simulink model "VIPStateCtrl"  (R2018b)
settings: Solver=FixedStepDiscrete  StartTime=0.0  StopTime=10.0  FixedStep=0.01  RelTol=1e-3
settings Model: Creator=sn2xws  LastModifiedBy=sn2xws
settings DataIOCC: SaveFormat=StructureWithTime
settings OptimizationCC: DefaultParameterBehavior=Inlined  EnhancedBackFolding=on  PassReuseOutputArgsAs=Individual arguments  ZeroExternalMemoryAtStartup=off  ZeroInternalMemoryAtStartup=off  OptimizeBlockOrder=speed  DifferentSizesBufferReuse=on  OptimizationCustomize=off
settings DebuggingCC: ParameterTunabilityLossMsg=error
settings ModelReferenceCC: ModelReferenceNumInstancesAllowed=Single
settings SFSimCC: MATLABDynamicMemAlloc=off
settings RTWCC: SystemTargetFile=autosar.tlc  GenCodeOnly=on  TemplateMakefile=ert_default_tmf  Description=AUTOSAR  GenerateReport=on  IncludeHyperlinkInReport=on  LaunchReport=on  GenerateTraceInfo=on  GenerateTraceReport=on  GenerateTraceReportSl=on  GenerateTraceReportSf=on  GenerateTraceReportEml=on
settings CodeAppCC: ForceParamTrailComments=on  IgnoreCustomStorageClasses=off  OperatorAnnotations=on  SimulinkDataObjDesc=on  SFDataObjDesc=on  InsertBlockDesc=on
settings STFCustomTargetCC: TargetLangStandard=C99 (ISO)  MultiwordLength=256  ParMdlRefBuildCompliant=on  CompOptLevelCompliant=on  IncludeMdlTerminateFcn=off  CombineOutputUpdateFcns=on  SuppressErrorStatus=on  ERTCustomFileBanners=on  SupportNonFinite=off  SupportComplex=off  SupportContinuousTime=off  SupportNonInlinedSFcns=off  RemoveResetFunc=on  MATLABClassNameForMDSCustomization=Simulink.SoftwareTarget.ERTCustomization  AutosarCompliant=on  UseToolchainInfoCompliant=on  LookupTableObjectStructAxisOrder=2,1,3,4,...  LUTObjectStructOrderEvenSpacing=Size,Table,Breakpoints  SystemTargetFile=autosar.tlc
settings ERTTargetCC: TargetLangStandard=C99 (ISO)  ConcurrentExecutionCompliant=off  IncludeMdlTerminateFcn=off  SuppressErrorStatus=on  SupportNonFinite=off  SupportComplex=off  ModelStepFunctionPrototypeControlCompliant=off  CPPClassGenCompliant=off  AutosarCompliant=on  LookupTableObjectStructAxisOrder=2,1,3,4,...  LUTObjectStructOrderEvenSpacing=Size,Table,Breakpoints  InlinedParameterPlacement=NonHierarchical  ERTCustomFileTemplate=example_file_process.tlc

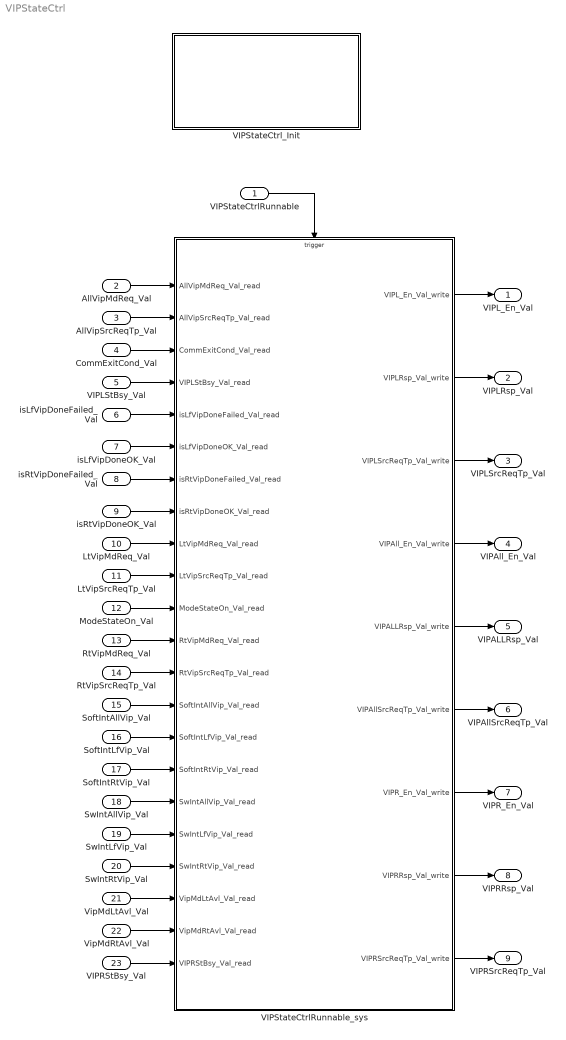
== system VIPStateCtrl ==
  VIPStateCtrlRunnable : Inport  SampleTime=0.01  OutputFunctionCall=on
  AllVipMdReq_Val : Inport  Port=2  OutDataTypeStr=boolean  PortDimensions=1
  AllVipSrcReqTp_Val : Inport  Port=3  OutDataTypeStr=Enum: SrcReqTp1  PortDimensions=1
  CommExitCond_Val : Inport  Port=4  OutDataTypeStr=boolean  PortDimensions=1
  VIPLStBsy_Val : Inport  Port=5  OutDataTypeStr=boolean  PortDimensions=1
  isLfVipDoneFailed_Val : Inport  Port=6  OutDataTypeStr=boolean  PortDimensions=1
  isLfVipDoneOK_Val : Inport  Port=7  OutDataTypeStr=boolean  PortDimensions=1
  isRtVipDoneFailed_Val : Inport  Port=8  OutDataTypeStr=boolean  PortDimensions=1
  isRtVipDoneOK_Val : Inport  Port=9  OutDataTypeStr=boolean  PortDimensions=1
  LtVipMdReq_Val : Inport  Port=10  OutDataTypeStr=boolean  PortDimensions=1
  LtVipSrcReqTp_Val : Inport  Port=11  OutDataTypeStr=Enum: SrcReqTp1  PortDimensions=1
  ModeStateOn_Val : Inport  Port=12  OutDataTypeStr=boolean  PortDimensions=1
  RtVipMdReq_Val : Inport  Port=13  OutDataTypeStr=boolean  PortDimensions=1
  RtVipSrcReqTp_Val : Inport  Port=14  OutDataTypeStr=Enum: SrcReqTp1  PortDimensions=1
  SoftIntAllVip_Val : Inport  Port=15  OutDataTypeStr=IntEnable  PortDimensions=1
  SoftIntLfVip_Val : Inport  Port=16  OutDataTypeStr=IntEnable  PortDimensions=1
  SoftIntRtVip_Val : Inport  Port=17  OutDataTypeStr=IntEnable  PortDimensions=1
  SwIntAllVip_Val : Inport  Port=18  OutDataTypeStr=IntEnable  PortDimensions=1
  SwIntLfVip_Val : Inport  Port=19  OutDataTypeStr=IntEnable  PortDimensions=1
  SwIntRtVip_Val : Inport  Port=20  OutDataTypeStr=IntEnable  PortDimensions=1
  VipMdLtAvl_Val : Inport  Port=21  OutDataTypeStr=boolean  PortDimensions=1
  VipMdRtAvl_Val : Inport  Port=22  OutDataTypeStr=boolean  PortDimensions=1
  VIPRStBsy_Val : Inport  Port=23  OutDataTypeStr=boolean  PortDimensions=1
  VIPStateCtrlRunnable_sys : Subsystem
  VIPStateCtrl_Init : Subsystem
  VIPL_En_Val : Outport  OutDataTypeStr=boolean  PortDimensions=1
  VIPLRsp_Val : Outport  Port=2  OutDataTypeStr=Enum: MdRspLocal1  PortDimensions=1
  VIPLSrcReqTp_Val : Outport  Port=3  OutDataTypeStr=Enum: SrcReqTp1  PortDimensions=1
  VIPAll_En_Val : Outport  Port=4  OutDataTypeStr=boolean  PortDimensions=1
  VIPALLRsp_Val : Outport  Port=5  OutDataTypeStr=Enum: MdRspLocal1  PortDimensions=1
  VIPAllSrcReqTp_Val : Outport  Port=6  OutDataTypeStr=Enum: SrcReqTp1  PortDimensions=1
  VIPR_En_Val : Outport  Port=7  OutDataTypeStr=boolean  PortDimensions=1
  VIPRRsp_Val : Outport  Port=8  OutDataTypeStr=Enum: MdRspLocal1  PortDimensions=1
  VIPRSrcReqTp_Val : Outport  Port=9  OutDataTypeStr=Enum: SrcReqTp1  PortDimensions=1
  wires:
  AllVipMdReq_Val/1 -> VIPStateCtrlRunnable_sys/1(AllVipMdReq_Val_read)
  AllVipSrcReqTp_Val/1 -> VIPStateCtrlRunnable_sys/2(AllVipSrcReqTp_Val_read)
  CommExitCond_Val/1 -> VIPStateCtrlRunnable_sys/3(CommExitCond_Val_read)
  VIPLStBsy_Val/1 -> VIPStateCtrlRunnable_sys/4(VIPLStBsy_Val_read)
  isLfVipDoneFailed_Val/1 -> VIPStateCtrlRunnable_sys/5(isLfVipDoneFailed_Val_read)
  isLfVipDoneOK_Val/1 -> VIPStateCtrlRunnable_sys/6(isLfVipDoneOK_Val_read)
  isRtVipDoneFailed_Val/1 -> VIPStateCtrlRunnable_sys/7(isRtVipDoneFailed_Val_read)
  isRtVipDoneOK_Val/1 -> VIPStateCtrlRunnable_sys/8(isRtVipDoneOK_Val_read)
  LtVipMdReq_Val/1 -> VIPStateCtrlRunnable_sys/9(LtVipMdReq_Val_read)
  LtVipSrcReqTp_Val/1 -> VIPStateCtrlRunnable_sys/10(LtVipSrcReqTp_Val_read)
  ModeStateOn_Val/1 -> VIPStateCtrlRunnable_sys/11(ModeStateOn_Val_read)
  RtVipMdReq_Val/1 -> VIPStateCtrlRunnable_sys/12(RtVipMdReq_Val_read)
  RtVipSrcReqTp_Val/1 -> VIPStateCtrlRunnable_sys/13(RtVipSrcReqTp_Val_read)
  SoftIntAllVip_Val/1 -> VIPStateCtrlRunnable_sys/14(SoftIntAllVip_Val_read)
  SoftIntLfVip_Val/1 -> VIPStateCtrlRunnable_sys/15(SoftIntLfVip_Val_read)
  SoftIntRtVip_Val/1 -> VIPStateCtrlRunnable_sys/16(SoftIntRtVip_Val_read)
  SwIntAllVip_Val/1 -> VIPStateCtrlRunnable_sys/17(SwIntAllVip_Val_read)
  SwIntLfVip_Val/1 -> VIPStateCtrlRunnable_sys/18(SwIntLfVip_Val_read)
  SwIntRtVip_Val/1 -> VIPStateCtrlRunnable_sys/19(SwIntRtVip_Val_read)
  VipMdLtAvl_Val/1 -> VIPStateCtrlRunnable_sys/20(VipMdLtAvl_Val_read)
  VipMdRtAvl_Val/1 -> VIPStateCtrlRunnable_sys/21(VipMdRtAvl_Val_read)
  VIPRStBsy_Val/1 -> VIPStateCtrlRunnable_sys/22(VIPRStBsy_Val_read)
  VIPStateCtrlRunnable_sys/1(VIPL_En_Val_write) -> VIPL_En_Val/1
  VIPStateCtrlRunnable_sys/2(VIPLRsp_Val_write) -> VIPLRsp_Val/1
  VIPStateCtrlRunnable_sys/3(VIPLSrcReqTp_Val_write) -> VIPLSrcReqTp_Val/1
  VIPStateCtrlRunnable_sys/4(VIPAll_En_Val_write) -> VIPAll_En_Val/1
  VIPStateCtrlRunnable_sys/5(VIPALLRsp_Val_write) -> VIPALLRsp_Val/1
  VIPStateCtrlRunnable_sys/6(VIPAllSrcReqTp_Val_write) -> VIPAllSrcReqTp_Val/1
  VIPStateCtrlRunnable_sys/7(VIPR_En_Val_write) -> VIPR_En_Val/1
  VIPStateCtrlRunnable_sys/8(VIPRRsp_Val_write) -> VIPRRsp_Val/1
  VIPStateCtrlRunnable_sys/9(VIPRSrcReqTp_Val_write) -> VIPRSrcReqTp_Val/1
  VIPStateCtrlRunnable/1 -> VIPStateCtrlRunnable_sys/Trigger

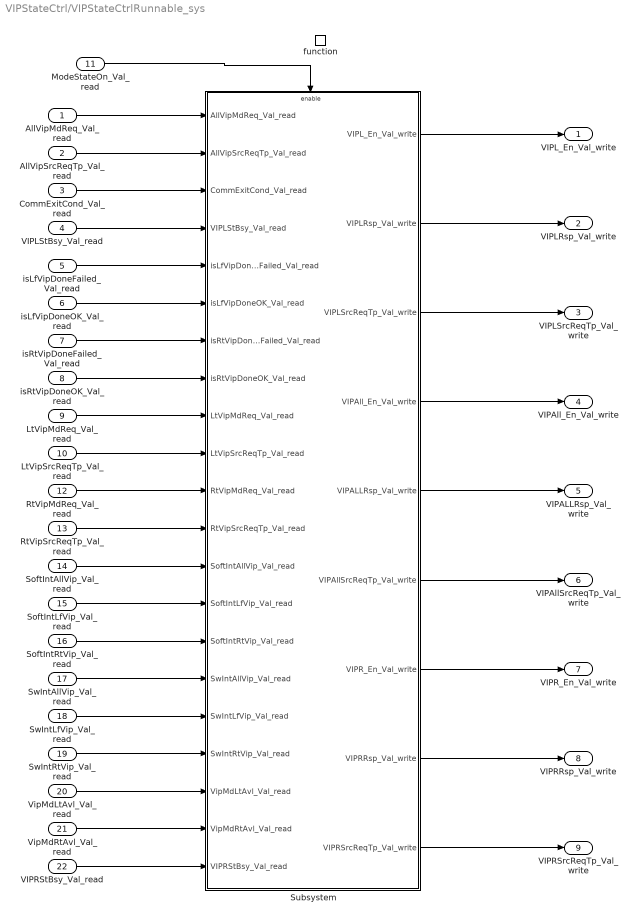
== system VIPStateCtrl/VIPStateCtrlRunnable_sys ==
  AllVipMdReq_Val_read : Inport
  AllVipSrcReqTp_Val_read : Inport  Port=2
  CommExitCond_Val_read : Inport  Port=3
  VIPLStBsy_Val_read : Inport  Port=4
  isLfVipDoneFailed_Val_read : Inport  Port=5
  isLfVipDoneOK_Val_read : Inport  Port=6
  isRtVipDoneFailed_Val_read : Inport  Port=7
  isRtVipDoneOK_Val_read : Inport  Port=8
  LtVipMdReq_Val_read : Inport  Port=9
  LtVipSrcReqTp_Val_read : Inport  Port=10
  ModeStateOn_Val_read : Inport  Port=11
  RtVipMdReq_Val_read : Inport  Port=12
  RtVipSrcReqTp_Val_read : Inport  Port=13
  SoftIntAllVip_Val_read : Inport  Port=14
  SoftIntLfVip_Val_read : Inport  Port=15
  SoftIntRtVip_Val_read : Inport  Port=16
  SwIntAllVip_Val_read : Inport  Port=17
  SwIntLfVip_Val_read : Inport  Port=18
  SwIntRtVip_Val_read : Inport  Port=19
  VipMdLtAvl_Val_read : Inport  Port=20
  VipMdRtAvl_Val_read : Inport  Port=21
  VIPRStBsy_Val_read : Inport  Port=22
  function : TriggerPort  TriggerType=function-call  VariantControl=(inherit)  SampleTimeType=periodic  SampleTime=-1
  Subsystem : Subsystem
  VIPL_En_Val_write : Outport
      settings: EnsureOutportIsVirtual=on
  VIPLRsp_Val_write : Outport  Port=2
      settings: EnsureOutportIsVirtual=on
  VIPLSrcReqTp_Val_write : Outport  Port=3
      settings: EnsureOutportIsVirtual=on
  VIPAll_En_Val_write : Outport  Port=4
      settings: EnsureOutportIsVirtual=on
  VIPALLRsp_Val_write : Outport  Port=5
      settings: EnsureOutportIsVirtual=on
  VIPAllSrcReqTp_Val_write : Outport  Port=6
      settings: EnsureOutportIsVirtual=on
  VIPR_En_Val_write : Outport  Port=7
      settings: EnsureOutportIsVirtual=on
  VIPRRsp_Val_write : Outport  Port=8
      settings: EnsureOutportIsVirtual=on
  VIPRSrcReqTp_Val_write : Outport  Port=9
      settings: EnsureOutportIsVirtual=on
  wires:
  ModeStateOn_Val_read/1 -> Subsystem/Enable
  AllVipMdReq_Val_read/1 -> Subsystem/1(AllVipMdReq_Val_read)
  AllVipSrcReqTp_Val_read/1 -> Subsystem/2(AllVipSrcReqTp_Val_read)
  CommExitCond_Val_read/1 -> Subsystem/3(CommExitCond_Val_read)
  VIPLStBsy_Val_read/1 -> Subsystem/4(VIPLStBsy_Val_read)
  isLfVipDoneFailed_Val_read/1 -> Subsystem/5(isLfVipDoneFailed_Val_read)
  isLfVipDoneOK_Val_read/1 -> Subsystem/6(isLfVipDoneOK_Val_read)
  isRtVipDoneFailed_Val_read/1 -> Subsystem/7(isRtVipDoneFailed_Val_read)
  isRtVipDoneOK_Val_read/1 -> Subsystem/8(isRtVipDoneOK_Val_read)
  LtVipMdReq_Val_read/1 -> Subsystem/9(LtVipMdReq_Val_read)
  LtVipSrcReqTp_Val_read/1 -> Subsystem/10(LtVipSrcReqTp_Val_read)
  RtVipMdReq_Val_read/1 -> Subsystem/11(RtVipMdReq_Val_read)
  RtVipSrcReqTp_Val_read/1 -> Subsystem/12(RtVipSrcReqTp_Val_read)
  SoftIntAllVip_Val_read/1 -> Subsystem/13(SoftIntAllVip_Val_read)
  SoftIntLfVip_Val_read/1 -> Subsystem/14(SoftIntLfVip_Val_read)
  SoftIntRtVip_Val_read/1 -> Subsystem/15(SoftIntRtVip_Val_read)
  SwIntAllVip_Val_read/1 -> Subsystem/16(SwIntAllVip_Val_read)
  SwIntLfVip_Val_read/1 -> Subsystem/17(SwIntLfVip_Val_read)
  SwIntRtVip_Val_read/1 -> Subsystem/18(SwIntRtVip_Val_read)
  VipMdLtAvl_Val_read/1 -> Subsystem/19(VipMdLtAvl_Val_read)
  VipMdRtAvl_Val_read/1 -> Subsystem/20(VipMdRtAvl_Val_read)
  VIPRStBsy_Val_read/1 -> Subsystem/21(VIPRStBsy_Val_read)
  Subsystem/1(VIPL_En_Val_write) -> VIPL_En_Val_write/1
  Subsystem/2(VIPLRsp_Val_write) -> VIPLRsp_Val_write/1
  Subsystem/3(VIPLSrcReqTp_Val_write) -> VIPLSrcReqTp_Val_write/1
  Subsystem/4(VIPAll_En_Val_write) -> VIPAll_En_Val_write/1
  Subsystem/5(VIPALLRsp_Val_write) -> VIPALLRsp_Val_write/1
  Subsystem/6(VIPAllSrcReqTp_Val_write) -> VIPAllSrcReqTp_Val_write/1
  Subsystem/7(VIPR_En_Val_write) -> VIPR_En_Val_write/1
  Subsystem/8(VIPRRsp_Val_write) -> VIPRRsp_Val_write/1
  Subsystem/9(VIPRSrcReqTp_Val_write) -> VIPRSrcReqTp_Val_write/1

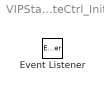
== system VIPStateCtrl/VIPStateCtrl_Init ==
  Event Listener : EventListener  EventName=reset

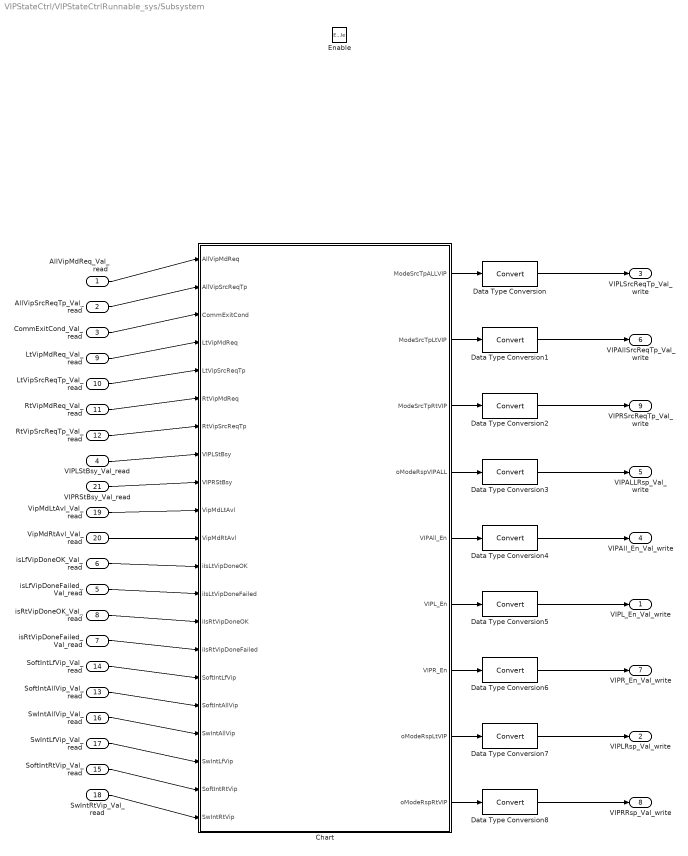
== system VIPStateCtrl/VIPStateCtrlRunnable_sys/Subsystem ==
  AllVipMdReq_Val_read : Inport
  AllVipSrcReqTp_Val_read : Inport  Port=2
  CommExitCond_Val_read : Inport  Port=3
  VIPLStBsy_Val_read : Inport  Port=4
  isLfVipDoneFailed_Val_read : Inport  Port=5
  isLfVipDoneOK_Val_read : Inport  Port=6
  isRtVipDoneFailed_Val_read : Inport  Port=7
  isRtVipDoneOK_Val_read : Inport  Port=8
  LtVipMdReq_Val_read : Inport  Port=9
  LtVipSrcReqTp_Val_read : Inport  Port=10
  RtVipMdReq_Val_read : Inport  Port=11
  RtVipSrcReqTp_Val_read : Inport  Port=12
  SoftIntAllVip_Val_read : Inport  Port=13
  SoftIntLfVip_Val_read : Inport  Port=14
  SoftIntRtVip_Val_read : Inport  Port=15
  SwIntAllVip_Val_read : Inport  Port=16
  SwIntLfVip_Val_read : Inport  Port=17
  SwIntRtVip_Val_read : Inport  Port=18
  VipMdLtAvl_Val_read : Inport  Port=19
  VipMdRtAvl_Val_read : Inport  Port=20
  VIPRStBsy_Val_read : Inport  Port=21
  Enable : EnablePort
  Chart : Stateflow chart  TreatAsAtomicUnit=on
  Data Type Conversion{,1..8} (9 alike) : DataTypeConversion
  VIPL_En_Val_write : Outport
  VIPLRsp_Val_write : Outport  Port=2
  VIPLSrcReqTp_Val_write : Outport  Port=3
  VIPAll_En_Val_write : Outport  Port=4
  VIPALLRsp_Val_write : Outport  Port=5
  VIPAllSrcReqTp_Val_write : Outport  Port=6
  VIPR_En_Val_write : Outport  Port=7
  VIPRRsp_Val_write : Outport  Port=8
  VIPRSrcReqTp_Val_write : Outport  Port=9
  wires:
  Chart/6(VIPL_En) -> Data Type Conversion5/1
  Chart/7(VIPR_En) -> Data Type Conversion6/1
  Chart/9(oModeRspRtVIP) -> Data Type Conversion8/1
  Chart/8(oModeRspLtVIP) -> Data Type Conversion7/1
  Chart/5(VIPAll_En) -> Data Type Conversion4/1
  Chart/3(ModeSrcTpRtVIP) -> Data Type Conversion2/1
  Chart/2(ModeSrcTpLtVIP) -> Data Type Conversion1/1
  Chart/4(oModeRspVIPALL) -> Data Type Conversion3/1
  Chart/1(ModeSrcTpALLVIP) -> Data Type Conversion/1
  AllVipMdReq_Val_read/1 -> Chart/1(AllVipMdReq)
  AllVipSrcReqTp_Val_read/1 -> Chart/2(AllVipSrcReqTp)
  CommExitCond_Val_read/1 -> Chart/3(CommExitCond)
  LtVipMdReq_Val_read/1 -> Chart/4(LtVipMdReq)
  LtVipSrcReqTp_Val_read/1 -> Chart/5(LtVipSrcReqTp)
  RtVipMdReq_Val_read/1 -> Chart/6(RtVipMdReq)
  RtVipSrcReqTp_Val_read/1 -> Chart/7(RtVipSrcReqTp)
  VIPLStBsy_Val_read/1 -> Chart/8(VIPLStBsy)
  VIPRStBsy_Val_read/1 -> Chart/9(VIPRStBsy)
  VipMdLtAvl_Val_read/1 -> Chart/10(VipMdLtAvl)
  VipMdRtAvl_Val_read/1 -> Chart/11(VipMdRtAvl)
  isLfVipDoneOK_Val_read/1 -> Chart/12(iIsLtVipDoneOK)
  isLfVipDoneFailed_Val_read/1 -> Chart/13(iIsLtVipDoneFailed)
  isRtVipDoneOK_Val_read/1 -> Chart/14(iIsRtVipDoneOK)
  isRtVipDoneFailed_Val_read/1 -> Chart/15(iIsRtVipDoneFailed)
  SoftIntLfVip_Val_read/1 -> Chart/16(SoftIntLfVip)
  SoftIntAllVip_Val_read/1 -> Chart/17(SoftIntAllVip)
  SwIntAllVip_Val_read/1 -> Chart/18(SwIntAllVip)
  SwIntLfVip_Val_read/1 -> Chart/19(SwIntLfVip)
  SoftIntRtVip_Val_read/1 -> Chart/20(SoftIntRtVip)
  SwIntRtVip_Val_read/1 -> Chart/21(SwIntRtVip)
  Data Type Conversion/1 -> VIPLSrcReqTp_Val_write/1
  Data Type Conversion1/1 -> VIPAllSrcReqTp_Val_write/1
  Data Type Conversion2/1 -> VIPRSrcReqTp_Val_write/1
  Data Type Conversion3/1 -> VIPALLRsp_Val_write/1
  Data Type Conversion4/1 -> VIPAll_En_Val_write/1
  Data Type Conversion5/1 -> VIPL_En_Val_write/1
  Data Type Conversion6/1 -> VIPR_En_Val_write/1
  Data Type Conversion7/1 -> VIPLRsp_Val_write/1
  Data Type Conversion8/1 -> VIPRRsp_Val_write/1

== stateflow chart VIPStateCtrl/VIPStateCtrlRunnable_sys/Subsystem/Chart ==
  state VIPStateCtrl
    state VIPL [parallel]
      settings: executionOrder=1
      state VIPLIlde
        en:VIPL_En = 0;
        en:ModeSrcTpLtVIP=SrcReqTp1.SrcReqTp_None;
        en:ChkVIPAll();
      state VIPLtOngoing
        en:VIPL_En = 1;
        en:ModeSrcTpALLVIP =AllVipSrcReqTp;
        en:oModeRspLtVIP = MdRsp_RecallOngoing;
      (default) -> VIPLIlde
      VIPLIlde -> VIPLtOngoing [order 1] : [(AllVipMdReq)&& VIPLStBsy ==0&&VipMdLtAvl==1 ]
          | {VIPAll_En =1;oModeRspVIPALL =MdRsp_RecallOngoing;ModeSrcTpLtVIP=AllVipSrcReqTp;}
      VIPLIlde -> VIPLtOngoing [order 2] : [(LtVipMdReq)&& VIPLStBsy ==0]{ModeSrcTpLtVIP = LtVipSrcReqTp;}
      VIPLtOngoing -> VIPLIlde [order 1] : [hasChangedTo(SoftIntLfVip,true)...
          | ||((hasChangedTo(SoftIntAllVip,true)||hasChangedTo(SwIntAllVip,true))&&VIPAll_En)]{oModeRspLtVIP = MdRsp_RecallUnsuccessfully_LocalInterrupt; }
      VIPLtOngoing -> VIPLIlde [order 2] : [hasChangedTo(SwIntLfVip,true)]{oModeRspLtVIP = MdRsp_RecallUnsuccessfully_LocalInterrupt;}
      VIPLtOngoing -> VIPLIlde [order 3] : [hasChangedTo(iIsLtVipDoneOK,true)]{oModeRspLtVIP = MdRsp_RecallSuccessfully;}
      VIPLtOngoing -> VIPLIlde [order 4] : [CommExitCond]{oModeRspLtVIP = MdRsp_RecallUnsuccessfully_Error;}
      VIPLtOngoing -> VIPLIlde [order 5] : [hasChangedTo(iIsLtVipDoneFailed,true)]{oModeRspLtVIP = MdRsp_RecallUnsuccessfully_Error;}
    state VIPR [parallel]
      settings: executionOrder=2
      state VIPRtOngoing
        en:VIPR_En = 1;
        en:ModeSrcTpALLVIP =AllVipSrcReqTp;
        en:oModeRspRtVIP = MdRsp_RecallOngoing;
      state VIPRIdle
        en:VIPR_En = 0;
        en:ModeSrcTpRtVIP=SrcReqTp1.SrcReqTp_None;
        en:ChkVIPAll();
      (default) -> VIPRIdle
      VIPRIdle -> VIPRtOngoing [order 1] : [(AllVipMdReq)&&VIPRStBsy ==0&&VipMdRtAvl==1 ]
          | {VIPAll_En = 1;oModeRspVIPALL =MdRsp_RecallOngoing;ModeSrcTpRtVIP=AllVipSrcReqTp;}
      VIPRIdle -> VIPRtOngoing [order 2] : [(RtVipMdReq)&&VIPRStBsy ==0]{ModeSrcTpRtVIP = RtVipSrcReqTp;}
      VIPRtOngoing -> VIPRIdle [order 1] : [hasChangedTo(SoftIntRtVip,true)...
          | ||((hasChangedTo(SoftIntAllVip,true)||hasChangedTo(SwIntAllVip,true))&&VIPAll_En)]{oModeRspRtVIP = MdRsp_RecallUnsuccessfully_LocalInterrupt;}
      VIPRtOngoing -> VIPRIdle [order 2] : [hasChangedTo(SwIntRtVip,true)]{oModeRspRtVIP = MdRsp_RecallUnsuccessfully_LocalInterrupt; }
      VIPRtOngoing -> VIPRIdle [order 3] : [hasChangedTo(iIsRtVipDoneOK,true)]{oModeRspRtVIP = MdRsp_RecallSuccessfully}
      VIPRtOngoing -> VIPRIdle [order 4] : [CommExitCond]{oModeRspRtVIP = MdRsp_RecallUnsuccessfully_Error;}
      VIPRtOngoing -> VIPRIdle [order 5] : [hasChangedTo(iIsRtVipDoneFailed,true)]{oModeRspRtVIP = MdRsp_RecallUnsuccessfully_Error}
  state ChkVIPAll [function]
    (default) -> (junction 2)
    (junction 2) -> (junction 3) [order 1] : [VIPAll_En ==1&&VIPL_En==0&&VIPR_En==0]
    (junction 3) -> (junction 4) [order 1] : [VipMdLtAvl==VipMdRtAvl && oModeRspLtVIP ==oModeRspRtVIP]
    (junction 2) -> (junction 5) [order 2]
    (junction 3) -> (junction 6) [order 2] : {
        | VIPAll_En=0;
        | oModeRspVIPALL =MdRsp_RecallUnsuccessfully_Error;
        | ModeSrcTpALLVIP=SrcReqTp1.SrcReqTp_None;
        | }
    (junction 4) -> (junction 7) : {
        | VIPAll_En = 0;
        | oModeRspVIPALL =oModeRspLtVIP;
        | ModeSrcTpALLVIP =  SrcReqTp1.SrcReqTp_None;
        | }
    (junction 6) -> (junction 5)
    (junction 7) -> (junction 6)
  (default) -> VIPStateCtrl
  data: AllVipMdReq input; AllVipSrcReqTp input; CommExitCond input; LtVipMdReq input; LtVipSrcReqTp input; RtVipMdReq input; RtVipSrcReqTp input; VIPLStBsy input; VIPRStBsy input; VipMdLtAvl input; VipMdRtAvl input; ModeSrcTpALLVIP output Enum:SrcReqTp1; ModeSrcTpLtVIP output Enum:SrcReqTp1; ModeSrcTpRtVIP output Enum:SrcReqTp1; oModeRspVIPALL output Enum:MdRspLocal1; VIPAll_En output boolean; VIPL_En output boolean; VIPR_En output boolean; oModeRspLtVIP output Enum:MdRspLocal1; oModeRspRtVIP output Enum:MdRspLocal1; iIsLtVipDoneOK input; iIsLtVipDoneFailed input; iIsRtVipDoneOK input; iIsRtVipDoneFailed input; SoftIntLfVip input; SoftIntAllVip input; SwIntAllVip input; SwIntLfVip input; SoftIntRtVip input; SwIntRtVip input
